simulink model "sb13_3b"  (Simulink 6.0)
settings: Solver=ode45  SolverMode=SingleTasking  StartTime=0.0  StopTime=999999  MaxStep=10  RelTol=1e-3  AbsTol=1e-6
values from neighbouring files (symbols this model uses):
  Gs = 10/(60*s+1)/(.1*s+1)    [m0108d.m]    (also in m0109b.m = 1/(8*s+1)^3; m0113c.m = 180/(.2*s+1)^3; m0251.m = b0/(a2*s^2+a1*s+a0); m0252.m = b0/(a2*s^2+a1*s+a0))
  Kpr = 10    [m0108d.m]    (also in m0109b.m = 1; m0113c.m; m0404Bsp.m = 3)
  wdach = 0    [m0109b.m]    (also in m0404Bsp.m = 1)
  zdach = -.3    (= -0.3)    [m0109b.m]    (also in m0404Bsp.m = 1)
settings Model: LastModifiedBy=Froriep
settings DataIOCC: LimitDataPoints=off  SaveOutput=off  SaveTime=off
settings OptimizationCC: BooleanDataType=off
settings DebuggingCC: SolverPrmCheckMsg=none
settings HardwareCC: TargetUnknown=on

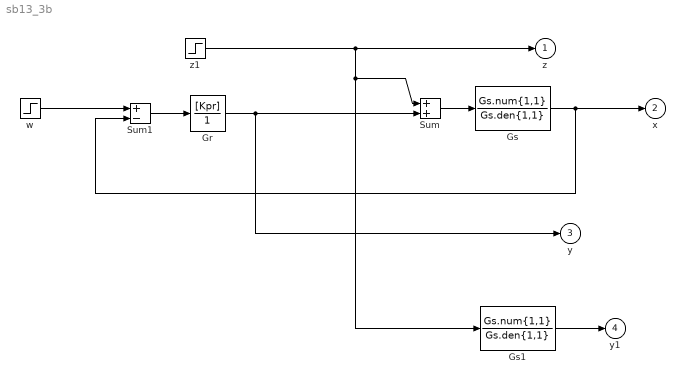
== system sb13_3b ==
  Gr : TransferFcn  Numerator=[Kpr]  Denominator=[1]
  Gs : TransferFcn  Numerator=Gs.num{1,1}  Denominator=Gs.den{1,1}
  Gs1 : TransferFcn  Numerator=Gs.num{1,1}  Denominator=Gs.den{1,1}
  Sum : Sum  SaturateOnIntegerOverflow=on  InputSameDT=on
  Sum1 : Sum  Inputs=+-  SaturateOnIntegerOverflow=on  InputSameDT=on
  w : Step  After=wdach  SampleTime=0
  z1 : Step  Time=10  After=zdach  SampleTime=0
  z : Outport  InitialOutput=0
  x : Outport  Port=2  InitialOutput=0
  y : Outport  Port=3  InitialOutput=0
  y1 : Outport  Port=4  InitialOutput=0
  wires:
  Gr/1 -> y/1, Sum/2
  Sum1/1 -> Gr/1
  w/1 -> Sum1/1
  Gs/1 -> Sum1/2, x/1
  z1/1 -> z/1, Sum/1, Gs1/1
  Sum/1 -> Gs/1
  Gs1/1 -> y1/1
